simulink model "hapticForceCtrlr_hack"  (R2025b)
settings: Solver=FixedStepAuto  StartTime=0.0  StopTime=inf  RelTol=1e-3  EnableMultiTasking=on
libraries: slpidlib x2
settings Model: SimulationMode=external  ExtModeTrigDuration=2  Creator=jyd1kor  LastModifiedBy=jyd1kor
settings SolverCC: AlgebraicLoopSolver=TrustRegion  PositivePriorityOrder=on
settings DataIOCC: ReturnWorkspaceOutputs=off
settings OptimizationCC: MaxStackSize=200000
settings DebuggingCC: ParameterTunabilityLossMsg=error  UnconnectedInputMsg=warning  UnconnectedOutputMsg=warning  UnconnectedLineMsg=warning  SubsystemReferenceDiagnosticForUnitTest=warning  ArithmeticOperatorsInVariantConditions=warning
settings HardwareCC: ProdBitPerLong=64.0  ProdLargestAtomicInteger=LongLong  ProdLargestAtomicFloat=Double  ProdLongLongMode=on  ProdHWDeviceType=ARM Compatible->ARM Cortex-A (64-bit)  UseEmbeddedCoderFeatures=off
settings ModelReferenceCC: EnableRefExpFcnMdlSchedulingChecks=on
settings SFSimCC: SimUseLocalCustomCode=off  CustomCodeUndefinedFunction=UseInterfaceOnly  SimTargetLang=C++  SimDLTargetLibrary=mkl-dnn
settings SFSimCC: SimCustomHeaderCode=|
  | da_connector.h
  | kuksa_bridge.h
settings SFSimCC: SimUserSources=|
  | da_connector.cpp
  | client.cpp
  | local/protogen/kuksa/val/v1/types.pb.cpp
  | local/protogen/kuksa/val/v1/types.grpc.pb.cpp
  | local/protogen/kuksa/val/v1/val.pb.cpp
  | local/protogen/kuksa/val/v1/val.grpc.pb.cpp
settings SFSimCC: SimUserIncludeDirs=|
  | local/protogen/kuksa/val/v1/
  | /lib/x86_64-linux-gnu
settings SFSimCC: SimUserLibraries=|
  | libgrpc++.so
  | libgrpc.so
  | libgpr.so
  | libprotobuf.so
  | libaddress_sorting.so
  | libre2.so
  | libupb.so
  | libcares.so
  | libz.so
  | libssl.so
  | libcrypto.so
  | libabsl_synchronization.so
  | libabsl_base.so
  | libabsl_time.so
  | libabsl_strings.so
  | libabsl_strings_internal.so
  | libabsl_str_format_internal.so
  | libabsl_cord.so
  | libabsl_cordz_info.so
  | libabsl_cord_internal.so
  | libabsl_cordz_functions.so
  | libabsl_cordz_handle.so
  | libabsl_exponential_biased.so
  | libabsl_stacktrace.so
  | libabsl_symbolize.so
  | libabsl_debugging_internal.so
  | libabsl_demangle_internal.so
  | libabsl_malloc_internal.so
  | libabsl_graphcycles_internal.so
  | libabsl_spinlock_wait.so
  | libabsl_int128.so
  | libabsl_throw_delegate.so
  | libabsl_raw_logging_internal.so
  | libabsl_log_severity.so
  | libabsl_civil_time.so
  | libabsl_time_zone.so
  | libabsl_hash.so
  | libabsl_city.so
  | libabsl_low_level_hash.so
  | libabsl_hashtablez_sampler.so
  | libabsl_raw_hash_set.so
  | libabsl_status.so
  | libabsl_statusor.so
  | libabsl_strerror.so
  | libabsl_bad_optional_access.so
  | libabsl_bad_variant_access.so
  | libabsl_random_distributions.so
  | libabsl_random_seed_sequences.so
  | libabsl_random_internal_pool_urbg.so
  | libabsl_random_internal_randen.so
  | libabsl_random_internal_randen_hwaes.so
  | libabsl_random_internal_randen_hwaes_impl.so
  | libabsl_random_internal_randen_slow.so
  | libabsl_random_internal_platform.so
  | libabsl_random_internal_seed_material.so
  | libabsl_random_seed_gen_exception.so
  | libpthread.so.0
  | libdl.so.2
  | librt.so.1
  | libatomic.so.1
settings RTWCC: SystemTargetFile=ert.tlc  HardwareBoard=Raspberry Pi (64bit)  TLCOptions="-aInlineSetEventsForThisBaseRateFcn=TLC_FALSE -aSuppressMultiTaskScheduler=TLC_FALSE  -aRateBasedStepFcn=0"  TemplateMakefile=ert_default_tmf  GenerateReport=on  RTWUseLocalCustomCode=off  CustomHeaderCode=da_connector.h  CustomSource=da_connector.c  Toolchain=GNU GCC Embedded Linux  BuildConfiguration=Faster Runs  LaunchReport=on  GPUComputeCapability=3.5  Description=Embedded Coder
settings CodeAppCC: ForceParamTrailComments=on  OperatorAnnotations=on  StateflowObjectComments=on  MATLABSourceComments=on
settings ERTTargetCC: ExtModeTransport=2.0  ExtModeStaticAlloc=on  ExtModeMexFile=ext_xcp  ExtModeIntrfLevel=Level2 - Open  InlinedParameterPlacement=Hierarchical  DynamicArrayContainerType=coder::array  ERTCustomFileBanners=off  SupportContinuousTime=on  SupportNonInlinedSFcns=on  RemoveResetFunc=off  SupportVariableSizeSignals=on  ModelStepFunctionPrototypeControlCompliant=off

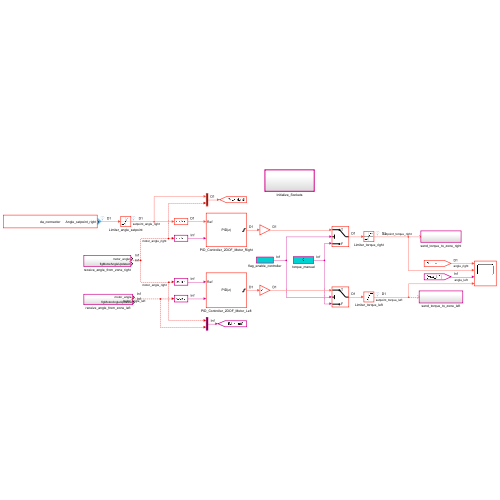
[thumbnail: Simulink's stored preview of the top-level diagram]
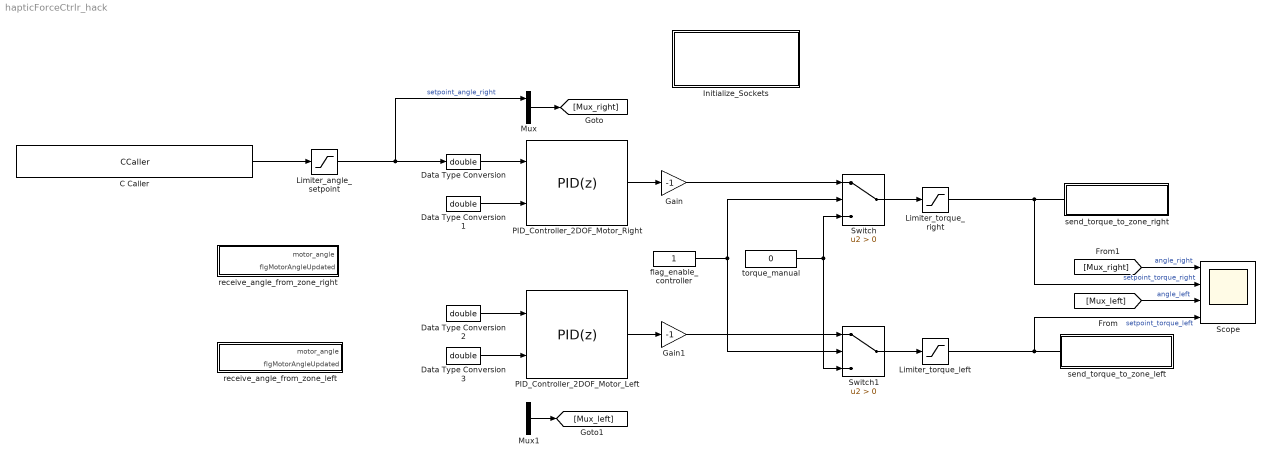
== system hapticForceCtrlr_hack ==
  C Caller : CCaller  FunctionName=da_connector  PortSpecificationStruct="%)30     .    , (   8    (     @         %    \"     $    !     0         %  0 \"0    $    _    07)G3F%M90  4&]R=$YA;64 4V-O<&4     26YD97@     5'EP90      4VEZ90      27-';&]B86P   X    P    !@    @    $          4    (     0    ,    !         !   P!O=70 #@   $@    &    \"     0         !0    @    !    %     $         $    !0   !!;F=L95]S971P;VEN=%]R:6=H=      .    .     8    (    !          %    \"     $    &     0         0    !@   $]U='!U=   #@   #@    &    \"     8         !0    @    !     0    $         \"0    @               X    X    !@    @    $          4    (     0    8    !         !     &    9&]U8FQE   .    ,     8    (    !          %    \"     $    !     0         0  $ ,0    X    P    !@    @    ) @        4    (     0    $    !          (  0"  SampleTime=0.1
  Data Type Conversion{,1..3} (4 alike) : DataTypeConversion  OutDataTypeStr=double  SaturateOnIntegerOverflow=off  RndMeth=Floor
  Gain : Gain  Gain=-1  OutDataTypeStr=single
  Gain1 : Gain  Gain=-1  OutDataTypeStr=single
  Initialize_Sockets : Subsystem  TreatAsAtomicUnit=on
  Limiter_angle_setpoint : Saturate  UpperLimit=1000.0  LowerLimit=-1000.0
  Limiter_torque_left : Saturate  UpperLimit=10  LowerLimit=-10
  Limiter_torque_right : Saturate  UpperLimit=10  LowerLimit=-10
  Mux : Mux  Inputs=2
  Mux1 : Mux  Inputs=2
  PID_Controller_2DOF_Motor_Left : slpidlib/PID Controller (2DOF)  Controller=PID  Form=Ideal  TimeDomain=Discrete-time  UseExternalTs=off  SampleTime=-1  IntegratorMethod=Forward Euler  FilterMethod=Forward Euler  ControllerParametersSource=internal  P=0.03  I=0.04  UseKiTs=off  D=0.0001  UseExternalDerivativeSource=off  N=10  UseFilter=on  b=1  c=0.8  TunerSelectOption=Transfer Function Based (PID Tuner App)  InitialConditionSource=internal  InitialConditionForIntegrator=0  InitialConditionForFilter=0  DifferentiatorICPrevScaledInput=0  ExternalReset=none  TrackingMode=off  Kt=1  LimitOutput=on  SatLimitsSource=internal  UpperSaturationLimit=10.0  LowerSaturationLimit=-10.0  LinearizeAsGain=off  AntiWindupMode=clamping  Kb=1  LimitIntegrator=off  UpperIntegratorSaturationLimit=inf  LowerIntegratorSaturationLimit=-inf  POutMin=[]  POutMax=[]  IOutMin=[]  IOutMax=[]  DOutMin=[]  DOutMax=[]  NOutMin=[]  NOutMax=[]  bOutMin=[]  bOutMax=[]  cOutMin=[]  cOutMax=[]  SumOutMin=[]  SumOutMax=[]  SaturationOutMin=[]  SaturationOutMax=[]  PParamMin=[]  PParamMax=[]  IParamMin=[]  IParamMax=[]  DParamMin=[]  DParamMax=[]  NParamMin=[]  NParamMax=[]  bParamMin=[]  bParamMax=[]  cParamMin=[]  cParamMax=[]  KbParamMin=[]  KbParamMax=[]  KtParamMin=[]  KtParamMax=[]  KbOutMin=[]  KbOutMax=[]  KtOutMin=[]  KtOutMax=[]  IntegratorOutMin=[]  IntegratorOutMax=[]  FilterOutMin=[]  FilterOutMax=[]  SumI1OutMin=[]  SumI1OutMax=[]  SumI2OutMin=[]  SumI2OutMax=[]  SumI3OutMin=[]  SumI3OutMax=[]  SumI4OutMin=[]  SumI4OutMax=[]  SumDOutMin=[]  SumDOutMax=[]  Sum1OutMin=[]  Sum1OutMax=[]  Sum2OutMin=[]  Sum2OutMax=[]  Sum3OutMin=[]  Sum3OutMax=[]  DifferentiatorOutMin=[]  DifferentiatorOutMax=[]  FilterDiffOutCoefMin=[]  FilterDiffOutCoefMax=[]  ReciprocalOutMin=[]  ReciprocalOutMax=[]  SumDenOutMin=[]  SumDenOutMax=[]  SumNumOutMin=[]  SumNumOutMax=[]  DivideOutMin=[]  DivideOutMax=[]  UdiffTsProdOutMin=[]  UdiffTsProdOutMax=[]  NTsProdOutMin=[]  NTsProdOutMax=[]  UintegralTsProdOutMin=[]  UintegralTsProdOutMax=[]  UngainTsProdOutMin=[]  UngainTsProdOutMax=[]  ClampingZeroOutDataTypeStr=Inherit: Inherit via back propagation  ClampingZeroOutMin=[]  ClampingZeroOutMax=[]  FilterDenConstantOutDataTypeStr=Inherit: Inherit via back propagation  FilterDenConstantOutMin=[]  FilterDenConstantOutMax=[]  PCopyOutDataTypeStr=Inherit: Inherit via back propagation  PCopyOutMin=[]  PCopyOutMax=[]  NCopyOutDataTypeStr=Inherit: Inherit via back propagation  NCopyOutMin=[]  NCopyOutMax=[]  IntegratorContinuousStateAttributes=''  IntegratorStateMustResolveToSignalObject=off  IntegratorRTWStateStorageClass=Auto  FilterContinuousStateAttributes=''  FilterStateMustResolveToSignalObject=off  FilterRTWStateStorageClass=Auto  ParallelPVariant=Passthrough  IdealPVariant=InternalParameters  IVariant=InternalParameters  DVariant=InternalParameters  bVariant=InternalParameters  cVariant=InternalParameters  IntegratorVariant=Discrete  SatVariant=Enabled  AWVariant=DiscClampingIdeal  PCopyVariant=InternalParamsIdeal  TRVariant=Disabled  FdbkBlocksVariant=Forward  IdealPFdbkVariant=Disabled  SatFdbkVariant=Disabled  DerivativeFilterVariant=ForwardEulerFilter  NVariant=InternalParameters  NCopyVariant=Disabled  FilterICVariant=InternalICsFilter  IntegratorICVariant=InternalICs  ExternalResetVariant=Disabled  TRSumVariant=Passthrough  SumFdbkVariant=Disabled  SumVariant=Sum_PID  TsampFilterVariant=InternalTs  TsampNgainVariant=Passthrough  TsampIntegralVariant=Disabled_SignalSpec  ExternalSaturationOutDataTypeStr=Inherit: Same as second input  DerivativeSourceVariant=ErrorSignal  PreIntVariant=InternalPreInt
      settings: LibrarySourceBlock=simulink/Discrete/Discrete PID Controller (2DOF)
  PID_Controller_2DOF_Motor_Right : slpidlib/PID Controller (2DOF)  Controller=PID  Form=Ideal  TimeDomain=Discrete-time  UseExternalTs=off  SampleTime=-1  IntegratorMethod=Forward Euler  FilterMethod=Forward Euler  ControllerParametersSource=internal  P=0.03  I=0.04  UseKiTs=off  D=0.0001  UseExternalDerivativeSource=off  N=10  UseFilter=on  b=1  c=0.8  TunerSelectOption=Transfer Function Based (PID Tuner App)  InitialConditionSource=internal  InitialConditionForIntegrator=0  InitialConditionForFilter=0  DifferentiatorICPrevScaledInput=0  ExternalReset=none  TrackingMode=off  Kt=1  LimitOutput=on  SatLimitsSource=internal  UpperSaturationLimit=10.0  LowerSaturationLimit=-10.0  LinearizeAsGain=off  AntiWindupMode=clamping  Kb=1  LimitIntegrator=off  UpperIntegratorSaturationLimit=inf  LowerIntegratorSaturationLimit=-inf  POutMin=[]  POutMax=[]  IOutMin=[]  IOutMax=[]  DOutMin=[]  DOutMax=[]  NOutMin=[]  NOutMax=[]  bOutMin=[]  bOutMax=[]  cOutMin=[]  cOutMax=[]  SumOutMin=[]  SumOutMax=[]  SaturationOutMin=[]  SaturationOutMax=[]  PParamMin=[]  PParamMax=[]  IParamMin=[]  IParamMax=[]  DParamMin=[]  DParamMax=[]  NParamMin=[]  NParamMax=[]  bParamMin=[]  bParamMax=[]  cParamMin=[]  cParamMax=[]  KbParamMin=[]  KbParamMax=[]  KtParamMin=[]  KtParamMax=[]  KbOutMin=[]  KbOutMax=[]  KtOutMin=[]  KtOutMax=[]  IntegratorOutMin=[]  IntegratorOutMax=[]  FilterOutMin=[]  FilterOutMax=[]  SumI1OutMin=[]  SumI1OutMax=[]  SumI2OutMin=[]  SumI2OutMax=[]  SumI3OutMin=[]  SumI3OutMax=[]  SumI4OutMin=[]  SumI4OutMax=[]  SumDOutMin=[]  SumDOutMax=[]  Sum1OutMin=[]  Sum1OutMax=[]  Sum2OutMin=[]  Sum2OutMax=[]  Sum3OutMin=[]  Sum3OutMax=[]  DifferentiatorOutMin=[]  DifferentiatorOutMax=[]  FilterDiffOutCoefMin=[]  FilterDiffOutCoefMax=[]  ReciprocalOutMin=[]  ReciprocalOutMax=[]  SumDenOutMin=[]  SumDenOutMax=[]  SumNumOutMin=[]  SumNumOutMax=[]  DivideOutMin=[]  DivideOutMax=[]  UdiffTsProdOutMin=[]  UdiffTsProdOutMax=[]  NTsProdOutMin=[]  NTsProdOutMax=[]  UintegralTsProdOutMin=[]  UintegralTsProdOutMax=[]  UngainTsProdOutMin=[]  UngainTsProdOutMax=[]  ClampingZeroOutDataTypeStr=Inherit: Inherit via back propagation  ClampingZeroOutMin=[]  ClampingZeroOutMax=[]  FilterDenConstantOutDataTypeStr=Inherit: Inherit via back propagation  FilterDenConstantOutMin=[]  FilterDenConstantOutMax=[]  PCopyOutDataTypeStr=Inherit: Inherit via back propagation  PCopyOutMin=[]  PCopyOutMax=[]  NCopyOutDataTypeStr=Inherit: Inherit via back propagation  NCopyOutMin=[]  NCopyOutMax=[]  IntegratorContinuousStateAttributes=''  IntegratorStateMustResolveToSignalObject=off  IntegratorRTWStateStorageClass=Auto  FilterContinuousStateAttributes=''  FilterStateMustResolveToSignalObject=off  FilterRTWStateStorageClass=Auto  ParallelPVariant=Passthrough  IdealPVariant=InternalParameters  IVariant=InternalParameters  DVariant=InternalParameters  bVariant=InternalParameters  cVariant=InternalParameters  IntegratorVariant=Discrete  SatVariant=Enabled  AWVariant=DiscClampingIdeal  PCopyVariant=InternalParamsIdeal  TRVariant=Disabled  FdbkBlocksVariant=Forward  IdealPFdbkVariant=Disabled  SatFdbkVariant=Disabled  DerivativeFilterVariant=ForwardEulerFilter  NVariant=InternalParameters  NCopyVariant=Disabled  FilterICVariant=InternalICsFilter  IntegratorICVariant=InternalICs  ExternalResetVariant=Disabled  TRSumVariant=Passthrough  SumFdbkVariant=Disabled  SumVariant=Sum_PID  TsampFilterVariant=InternalTs  TsampNgainVariant=Passthrough  TsampIntegralVariant=Disabled_SignalSpec  ExternalSaturationOutDataTypeStr=Inherit: Same as second input  DerivativeSourceVariant=ErrorSignal  PreIntVariant=InternalPreInt
      settings: LibrarySourceBlock=simulink/Discrete/Discrete PID Controller (2DOF)
  Scope : Scope  NumInputPorts=4
      settings: ActiveDisplayYMinimum=-413.6462230682373  ActiveDisplayYMaximum=1342.9577617645264
  Switch : Switch  Criteria=u2 > Threshold  SaturateOnIntegerOverflow=off  InputSameDT=off
  Switch1 : Switch  Criteria=u2 > Threshold  SaturateOnIntegerOverflow=off  InputSameDT=off
  flag_enable_controller : Constant  OutDataTypeStr=boolean
  receive_angle_from_zone_left : Subsystem
  receive_angle_from_zone_right : Subsystem
  send_torque_to_zone_left : Subsystem
  send_torque_to_zone_right : Subsystem
  torque_manual : Constant  Value=0  OutDataTypeStr=single
  wires:
  Data Type Conversion3/1 -> PID_Controller_2DOF_Motor_Left/2
  [Mux_right] -> Scope/1  "angle_right"
  [Mux_left] -> Scope/3  "angle_left"
  Data Type Conversion/1 -> PID_Controller_2DOF_Motor_Right/1
  Mux/1 -> [Mux_right]
  torque_manual/1 -> Switch1/3, Switch/3
  Gain/1 -> Switch/1
  Switch1/1 -> Limiter_torque_left/1
  flag_enable_controller/1 -> Switch1/2, Switch/2
  PID_Controller_2DOF_Motor_Right/1 -> Gain/1
  Gain1/1 -> Switch1/1
  Limiter_torque_left/1 -> Scope/4  "setpoint_torque_left"
  ? -> Data Type Conversion3/1, Mux1/2  "motor_angle_left"
  Data Type Conversion2/1 -> PID_Controller_2DOF_Motor_Left/1
  Switch/1 -> Limiter_torque_right/1
  Limiter_torque_right/1 -> Scope/2  "setpoint_torque_right"
  PID_Controller_2DOF_Motor_Left/1 -> Gain1/1
  Limiter_angle_setpoint/1 -> Data Type Conversion/1, Mux/1  "setpoint_angle_right"
  Data Type Conversion1/1 -> PID_Controller_2DOF_Motor_Right/2
  Mux1/1 -> [Mux_left]
  ? -> Data Type Conversion2/1, Mux1/1, Data Type Conversion1/1, Mux/2  "motor_angle_right"
  C Caller/1 -> Limiter_angle_setpoint/1

== system hapticForceCtrlr_hack/Initialize_Sockets ==

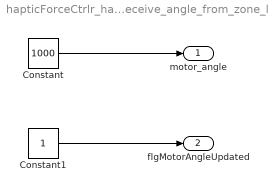
== system hapticForceCtrlr_hack/receive_angle_from_zone_left ==
  Constant : Constant  Value=1000  OutDataTypeStr=uint32
  Constant1 : Constant  OutDataTypeStr=boolean
  motor_angle : Outport
  flgMotorAngleUpdated : Outport  Port=2
  wires:
  Constant/1 -> motor_angle/1
  Constant1/1 -> flgMotorAngleUpdated/1

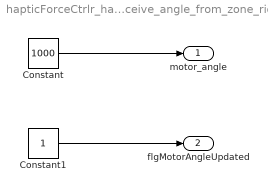
== system hapticForceCtrlr_hack/receive_angle_from_zone_right ==
  Constant : Constant  Value=1000  OutDataTypeStr=uint32
  Constant1 : Constant  OutDataTypeStr=boolean
  motor_angle : Outport
  flgMotorAngleUpdated : Outport  Port=2
  wires:
  Constant/1 -> motor_angle/1
  Constant1/1 -> flgMotorAngleUpdated/1

== system hapticForceCtrlr_hack/send_torque_to_zone_left ==

== system hapticForceCtrlr_hack/send_torque_to_zone_right ==
